simulink model "SistemaSeguimientoSinIntegrador"  (R2020a)
settings: Solver=VariableStepAuto  StartTime=0.0  StopTime=10  RelTol=1e-3
settings Model: Creator=Sergio  LastModifiedBy=Sergio

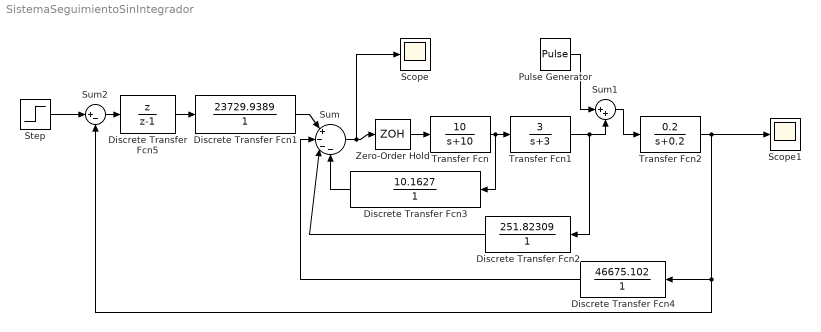
== system SistemaSeguimientoSinIntegrador ==
  Discrete Transfer Fcn1 : DiscreteTransferFcn  Numerator=[23729.9389]  Denominator=[1]
  Discrete Transfer Fcn2 : DiscreteTransferFcn  Numerator=[251.82309]  Denominator=[1]
  Discrete Transfer Fcn3 : DiscreteTransferFcn  Numerator=[10.1627]  Denominator=[1]
  Discrete Transfer Fcn4 : DiscreteTransferFcn  Numerator=[46675.102]  Denominator=[1]
  Discrete Transfer Fcn5 : DiscreteTransferFcn  Numerator=[1 0]  Denominator=[1 -1]
  Pulse Generator : DiscretePulseGenerator  PulseType=Time based  Amplitude=10  Period=10
  Scope : Scope
  Scope1 : Scope
  Step : Step  SampleTime=0
  Sum : Sum  Inputs=|+---
  Sum1 : Sum  Inputs=|++
  Sum2 : Sum  Inputs=|+-
  Transfer Fcn : TransferFcn  Numerator=[10]  Denominator=[1 10]
  Transfer Fcn1 : TransferFcn  Numerator=[3]  Denominator=[1 3]
  Transfer Fcn2 : TransferFcn  Numerator=[0.2]  Denominator=[1 0.2]
  Zero-Order Hold : ZeroOrderHold  SampleTime=0.02
  wires:
  Zero-Order Hold/1 -> Transfer Fcn/1
  Transfer Fcn/1 -> Discrete Transfer Fcn3/1, Transfer Fcn1/1
  Sum/1 -> Scope/1, Zero-Order Hold/1
  Transfer Fcn2/1 -> Discrete Transfer Fcn4/1, Sum2/2, Scope1/1
  Transfer Fcn1/1 -> Discrete Transfer Fcn2/1, Sum1/2
  Sum1/1 -> Transfer Fcn2/1
  Discrete Transfer Fcn3/1 -> Sum/4
  Discrete Transfer Fcn2/1 -> Sum/3
  Pulse Generator/1 -> Sum1/1
  Step/1 -> Sum2/1
  Discrete Transfer Fcn1/1 -> Sum/1
  Discrete Transfer Fcn5/1 -> Discrete Transfer Fcn1/1
  Sum2/1 -> Discrete Transfer Fcn5/1
  Discrete Transfer Fcn4/1 -> Sum/2
